simulink model "figure_1_12"  (R2026a)
settings: Solver=ode5  FixedStep=1e-4
undefined symbols (not defined in the file): J, k
settings Model: Creator=yagmu  LastModifiedBy=yagmu

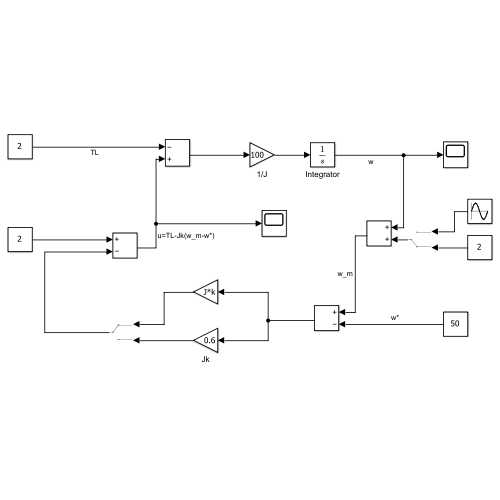
[thumbnail: Simulink's stored preview of the top-level diagram]
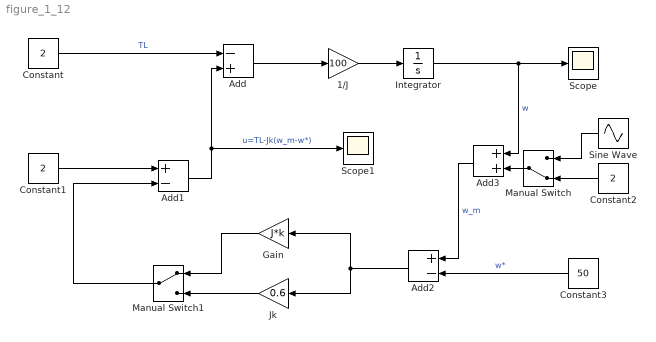
== system figure_1_12 ==
  1/J : Gain  Gain=100
  Add : Sum  Inputs=-+
  Add1 : Sum  Inputs=+-
  Add2 : Sum  Inputs=+-
  Add3 : Sum
  Constant : Constant  Value=2
  Constant1 : Constant  Value=2
  Constant2 : Constant  Value=2
  Constant3 : Constant  Value=50
  Gain : Gain  Gain=J*k
  Integrator : Integrator  InitialCondition=50
  Jk : Gain  Gain=0.6
  Manual Switch : ManualSwitch  CurrentSetting=0
  Manual Switch1 : ManualSwitch
  Scope : Scope
      settings: ActiveDisplayYMinimum=-207.64132472859478  ActiveDisplayYMaximum=157.29087852862156
  Scope1 : Scope
      settings: ActiveDisplayYMinimum=1.8875000000000441  ActiveDisplayYMaximum=2.0124999999996005
  Sine Wave : Sin  Amplitude=0.3  Frequency=24  SampleTime=0
  wires:
  Add/1 -> 1/J/1
  1/J/1 -> Integrator/1
  Integrator/1 -> Scope/1, Add3/1  "w"
  Add1/1 -> Add/2, Scope1/1  "u=TL-Jk(w_m-w*)"
  Manual Switch1/1 -> Add1/2
  Constant3/1 -> Add2/2  "w*"
  Gain/1 -> Manual Switch1/1
  Jk/1 -> Manual Switch1/2
  Add2/1 -> Jk/1, Gain/1
  Constant1/1 -> Add1/1
  Constant/1 -> Add/1  "TL"
  Sine Wave/1 -> Manual Switch/1
  Constant2/1 -> Manual Switch/2
  Manual Switch/1 -> Add3/2
  Add3/1 -> Add2/1  "w_m"
